simulink library "controlAllocation_cl"  (R2018b)
settings: Solver=VariableStepAuto  StartTime=0.0  StopTime=10.0  RelTol=1e-3
libraries: sharedutil x1
settings Model: Creator=James Reed  LastModifiedBy=James Reed

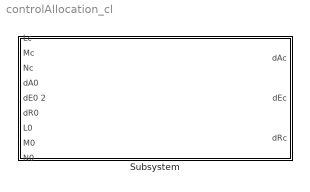
== system controlAllocation_cl ==
  Subsystem : Subsystem

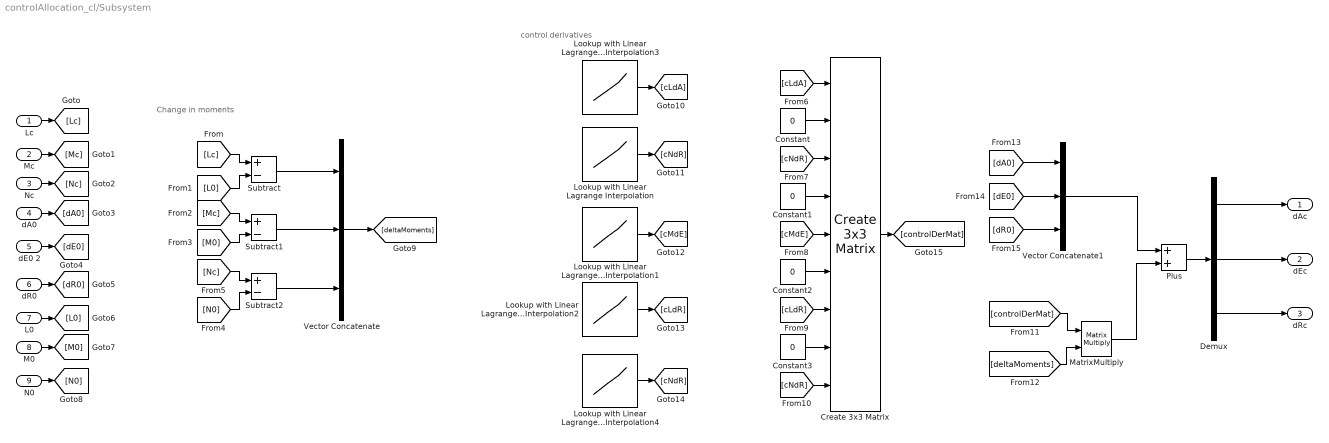
== system controlAllocation_cl/Subsystem ==
  note: control derivatives
  note: Change in moments
  Lc : Inport
  Mc : Inport  Port=2
  "Nc " : Inport  Port=3
  dA0 : Inport  Port=4
  dE0 2 : Inport  Port=5
  dR0 : Inport  Port=6
  L0 : Inport  Port=7
  M0 : Inport  Port=8
  N0 : Inport  Port=9
  Constant{,1..3} (4 alike) : Constant  Value=0
  Create 3x3 Matrix : sharedutil/Create 3x3 Matrix  aMode=aMode
  Demux : Demux  Outputs=3
  Lookup with Linear Lagrange Interpolation{,1..4} (5 alike) : Lookup_n-D  NumberOfTableDimensions=1  BreakpointsForDimension1=[-5:5]  Table=tanh([-5:5])  InterpMethod=Linear Lagrange  InternalRulePriority=Speed  RndMeth=Simplest  InputSameDT=on
  MatrixMultiply : Product  Multiplication=Matrix(*)
  Plus : Sum
  Subtract : Sum  Inputs=+-
  Subtract1 : Sum  Inputs=+-
  Subtract2 : Sum  Inputs=+-
  Vector Concatenate : Concatenate  NumInputs=3
  Vector Concatenate1 : Concatenate  NumInputs=3
  dAc : Outport
  "dEc " : Outport  Port=2
  "dRc " : Outport  Port=3
  wires:
  Constant/1 -> Create 3x3 Matrix/2
  Constant1/1 -> Create 3x3 Matrix/4
  Constant2/1 -> Create 3x3 Matrix/6
  Constant3/1 -> Create 3x3 Matrix/8
  Lc/1 -> [Lc]
  Mc/1 -> [Mc]
  "Nc "/1 -> [Nc]
  dA0/1 -> [dA0]
  dE0 2/1 -> [dE0]
  dR0/1 -> [dR0]
  L0/1 -> [L0]
  M0/1 -> [M0]
  N0/1 -> [N0]
  [Lc] -> Subtract/1
  [L0] -> Subtract/2
  [Mc] -> Subtract1/1
  [M0] -> Subtract1/2
  [N0] -> Subtract2/2
  [Nc] -> Subtract2/1
  Subtract1/1 -> Vector Concatenate/2
  Subtract/1 -> Vector Concatenate/1
  Subtract2/1 -> Vector Concatenate/3
  Vector Concatenate/1 -> [deltaMoments]
  Lookup with Linear Lagrange Interpolation3/1 -> [cLdA]
  Lookup with Linear Lagrange Interpolation/1 -> [cNdR]
  Lookup with Linear Lagrange Interpolation1/1 -> [cMdE]
  Lookup with Linear Lagrange Interpolation2/1 -> [cLdR]
  Lookup with Linear Lagrange Interpolation4/1 -> [cNdR]
  [cLdA] -> Create 3x3 Matrix/1
  [cNdR] -> Create 3x3 Matrix/3
  [cMdE] -> Create 3x3 Matrix/5
  [cLdR] -> Create 3x3 Matrix/7
  [cNdR] -> Create 3x3 Matrix/9
  Create 3x3 Matrix/1 -> [controlDerMat]
  [controlDerMat] -> MatrixMultiply/1
  [deltaMoments] -> MatrixMultiply/2
  MatrixMultiply/1 -> Plus/2
  [dR0] -> Vector Concatenate1/3
  [dA0] -> Vector Concatenate1/1
  [dE0] -> Vector Concatenate1/2
  Vector Concatenate1/1 -> Plus/1
  Plus/1 -> Demux/1
  Demux/3 -> "dRc "/1
  Demux/1 -> dAc/1
  Demux/2 -> "dEc "/1
